simulink model "bille_synthese_2"  (R2019b)
settings: Solver=ode45  StartTime=0.0  StopTime=30  RelTol=1e-3  EnableMultiTasking=on
undefined symbols (not defined in the file): f, J, k, k1, k2, k3, kb, ki, kp, kpi, kv, lm, nm, r0, r1, r2, rm, sp1, Te, tii
settings Model: ExtModeTrigMode=oneshot  ExtModeArmWhenConnect=off  Creator=khennouh  LastModifiedBy=lukas
settings DataIOCC: SaveFormat=Array  SignalLoggingSaveFormat=ModelDataLogs  ReturnWorkspaceOutputs=off
settings OptimizationCC: BlockReduction=off  BooleanDataType=off
settings DebuggingCC: SaveWithParameterizedLinksMsg=none  UnderspecifiedInitializationDetection=Classic  MergeDetectMultiDrivingBlocksExec=none  SignalResolutionControl=TryResolveAllWithWarning  MultiTaskDSMMsg=warning  MultiTaskCondExecSysMsg=none  ArithmeticOperatorsInVariantConditions=warning
settings HardwareCC: TargetUnknown=on
settings ModelReferenceCC: PropagateSignalLabelsOutOfModel=off
settings SFSimCC: SimUseLocalCustomCode=off  CustomCodeUndefinedFunction=UseInterfaceOnly
settings RTWCC: RTWUseLocalCustomCode=off
settings CodeAppCC: StateflowObjectComments=on
settings GRTTargetCC: TargetLangStandard=C89/C90 (ANSI)  CombineOutputUpdateFcns=off  GRTInterface=on

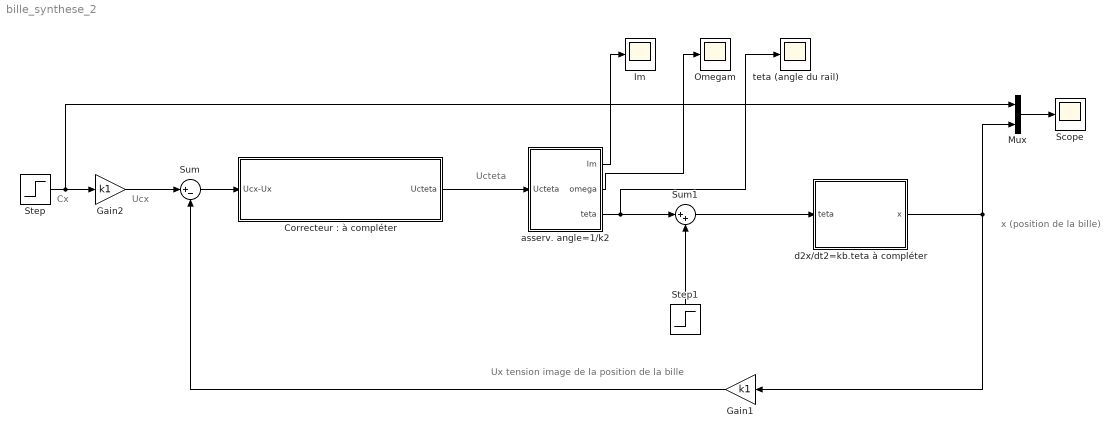
== system bille_synthese_2 ==
  note: Ucteta
  note: x (position de la bille)
  note: Ucx
  note: Ux tension image de la position de la bille
  note: Cx
  "Correcteur : à compléter" : Subsystem
  Gain1 : Gain  Gain=k1  SaturateOnIntegerOverflow=on  OutDataTypeStr=Inherit: Same as input  ParamDataTypeStr=Inherit: Same as input
  Gain2 : Gain  Gain=k1  SaturateOnIntegerOverflow=on  OutDataTypeStr=Inherit: Same as input  ParamDataTypeStr=Inherit: Same as input
  Im : Scope
  Mux : Mux  Inputs=2
  Omegam : Scope
  Scope : Scope
  Step : Step  After=0.1  SampleTime=0
  Step1 : Step  Time=10  After=1*pi/180  SampleTime=0
  Sum : Sum  Inputs=|+-  SaturateOnIntegerOverflow=on  InputSameDT=on  OutDataTypeStr=Inherit: Same as first input
  Sum1 : Sum  Inputs=|++  SaturateOnIntegerOverflow=on  InputSameDT=on  OutDataTypeStr=Inherit: Same as first input
  "asserv. angle=1/k2 " : Subsystem
  d2x/dt2=kb.teta à compléter : Subsystem
  teta (angle du rail) : Scope
  wires:
  "asserv. angle=1/k2 "/1(Im) -> Im/1
  "asserv. angle=1/k2 "/2(omega) -> Omegam/1
  Gain2/1 -> Sum/1
  Step/1 -> Mux/1, Gain2/1
  Step1/1 -> Sum1/2
  Mux/1 -> Scope/1
  "asserv. angle=1/k2 "/3(teta) -> teta (angle du rail)/1, Sum1/1
  d2x/dt2=kb.teta à compléter/1(x) -> Gain1/1, Mux/2
  Sum1/1 -> d2x/dt2=kb.teta à compléter/1(teta)
  Sum/1 -> "Correcteur : à compléter"/1(Ucx-Ux)
  "Correcteur : à compléter"/1(Ucteta) -> "asserv. angle=1/k2 "/1(Ucteta)
  Gain1/1 -> Sum/2

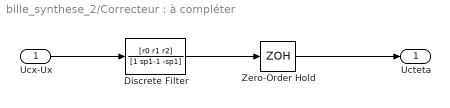
== system bille_synthese_2/Correcteur : à compléter ==
  Ucx-Ux : Inport
  Discrete Filter : DiscreteFilter  Numerator=[r0 r1 r2]  Denominator=[1 sp1-1 -sp1]  SampleTime=Te
  Zero-Order Hold : ZeroOrderHold  SampleTime=Te
  Ucteta : Outport  VectorParamsAs1DForOutWhenUnconnected=off
  wires:
  Ucx-Ux/1 -> Discrete Filter/1
  Zero-Order Hold/1 -> Ucteta/1
  Discrete Filter/1 -> Zero-Order Hold/1

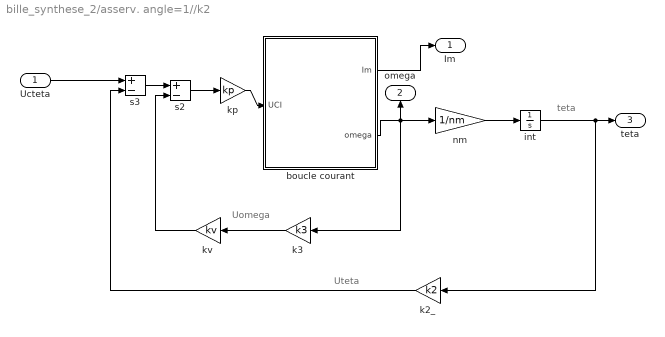
== system bille_synthese_2/asserv. angle=1//k2  ==
  note: Uomega
  note: teta
  note: Uteta
  Ucteta : Inport
  boucle courant : Subsystem
  int : Integrator
  k2_ : Gain  Gain=k2  SaturateOnIntegerOverflow=on  OutDataTypeStr=Inherit: Same as input  ParamDataTypeStr=Inherit: Same as input
  k3 : Gain  Gain=k3  SaturateOnIntegerOverflow=on  OutDataTypeStr=Inherit: Same as input  ParamDataTypeStr=Inherit: Same as input
  kp : Gain  Gain=kp  SaturateOnIntegerOverflow=on  OutDataTypeStr=Inherit: Same as input  ParamDataTypeStr=Inherit: Same as input
  kv : Gain  Gain=kv  SaturateOnIntegerOverflow=on  OutDataTypeStr=Inherit: Same as input  ParamDataTypeStr=Inherit: Same as input
  nm : Gain  Gain=1/nm  SaturateOnIntegerOverflow=on  OutDataTypeStr=Inherit: Same as input  ParamDataTypeStr=Inherit: Same as input
  s2 : Sum  Inputs=+-  SaturateOnIntegerOverflow=on  InputSameDT=on  OutDataTypeStr=Inherit: Same as first input
  s3 : Sum  Inputs=+-  SaturateOnIntegerOverflow=on  InputSameDT=on  OutDataTypeStr=Inherit: Same as first input
  Im : Outport  VectorParamsAs1DForOutWhenUnconnected=off
  omega : Outport  Port=2  VectorParamsAs1DForOutWhenUnconnected=off
  teta : Outport  Port=3  VectorParamsAs1DForOutWhenUnconnected=off
  wires:
  kp/1 -> boucle courant/1(UCI)
  s2/1 -> kp/1
  s3/1 -> s2/1
  nm/1 -> int/1
  boucle courant/2(omega) -> nm/1, k3/1, omega/1
  k3/1 -> kv/1
  kv/1 -> s2/2
  int/1 -> k2_/1, teta/1
  k2_/1 -> s3/2
  boucle courant/1(Im) -> Im/1
  Ucteta/1 -> s3/1

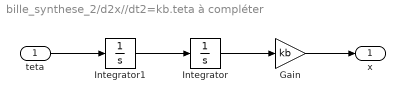
== system bille_synthese_2/d2x//dt2=kb.teta à compléter ==
  teta : Inport
  Gain : Gain  Gain=kb
  Integrator : Integrator
  Integrator1 : Integrator
  x : Outport  VectorParamsAs1DForOutWhenUnconnected=off
  wires:
  teta/1 -> Integrator1/1
  Integrator1/1 -> Integrator/1
  Integrator/1 -> Gain/1
  Gain/1 -> x/1

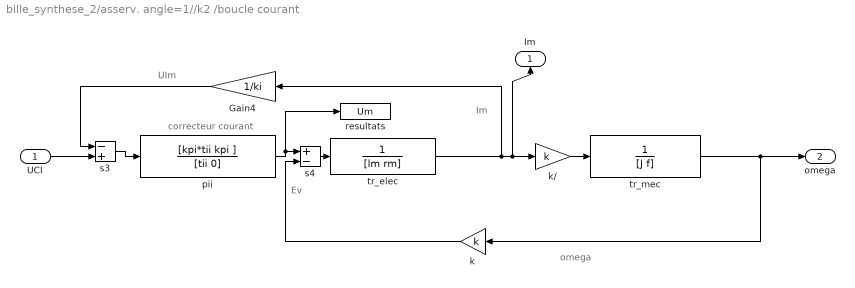
== system bille_synthese_2/asserv. angle=1//k2 /boucle courant ==
  note: correcteur courant
  note: Im
  note: Ev
  note: UIm
  note: omega
  UCI : Inport
  Gain4 : Gain  Gain=1/ki  SaturateOnIntegerOverflow=on  OutDataTypeStr=Inherit: Same as input  ParamDataTypeStr=Inherit: Same as input
  k : Gain  Gain=k  SaturateOnIntegerOverflow=on  OutDataTypeStr=Inherit: Same as input  ParamDataTypeStr=Inherit: Same as input
  "k/ " : Gain  Gain=k  SaturateOnIntegerOverflow=on  OutDataTypeStr=Inherit: Same as input  ParamDataTypeStr=Inherit: Same as input
  pii : TransferFcn  Numerator=[kpi*tii kpi ]  Denominator=[tii 0]
  resultats : ToWorkspace  VariableName=Um
      settings: MaxDataPoints=20000
  s3 : Sum  Inputs=-+  SaturateOnIntegerOverflow=on  InputSameDT=on  OutDataTypeStr=Inherit: Same as first input
  s4 : Sum  Inputs=+-  SaturateOnIntegerOverflow=on  InputSameDT=on  OutDataTypeStr=Inherit: Same as first input
  tr_elec : TransferFcn  Denominator=[lm rm]
  tr_mec : TransferFcn  Denominator=[J f]
  Im : Outport  VectorParamsAs1DForOutWhenUnconnected=off
  omega : Outport  Port=2  VectorParamsAs1DForOutWhenUnconnected=off
  wires:
  s4/1 -> tr_elec/1
  Gain4/1 -> s3/1
  s3/1 -> pii/1
  k/1 -> s4/2
  "k/ "/1 -> tr_mec/1
  tr_mec/1 -> k/1, omega/1
  UCI/1 -> s3/2
  pii/1 -> s4/1, resultats/1
  tr_elec/1 -> Gain4/1, "k/ "/1, Im/1
